simulink model "SixDOF_Equationgs_of_Motion"  (R2018a)
settings: Solver=VariableStepAuto  StartTime=0.0  StopTime=10  RelTol=1e-3
values from neighbouring files (symbols this model uses):
  CD0 = yD(find(~x))    [AOA_CL_CD_Cm.m]    (also in Linear_Coefficients.m = 0.051832)
  CDalpha = mean(diff(yD_linear)/d)    [AOA_CL_CD_Cm.m]    (also in Linear_Coefficients.m = 0.006587)
  CDdelta_e = 0.00036    [AOA_CL_CD_Cm.m]
  CL0 = yL(find(~x))    [AOA_CL_CD_Cm.m]    (also in Linear_Coefficients.m = 0.64791)
  CLalpha = mean(diff(yL_linear)/d)    [AOA_CL_CD_Cm.m]    (also in Linear_Coefficients.m = 0.088485)
  Clbeta = -0.00072    [AOA_CL_CD_Cm.m]    (also in Linear_Coefficients.m)
  Cldelta_a = -0.00393    [AOA_CL_CD_Cm.m]
  CLdelta_e = 0.00656    [AOA_CL_CD_Cm.m]    (also in Linear_Coefficients.m = 0.00328)
  Cldelta_r = -0.00008    (= -8e-05)    [AOA_CL_CD_Cm.m]
  Clp = -0.62    [AOA_CL_CD_Cm.m]    (also in Linear_Coefficients.m)
  Clr = -0.01    [AOA_CL_CD_Cm.m]    (also in Linear_Coefficients.m)
  Cm0 = ym(ZLI)    [AOA_CL_CD_Cm.m]    (also in Linear_Coefficients.m = -0.036061)
  Cmalpha = mean(diff(ym_linear)/d)    [AOA_CL_CD_Cm.m]    (also in Linear_Coefficients.m = -0.008902)
  Cmdelta_e = -0.01684    [AOA_CL_CD_Cm.m]    (also in Linear_Coefficients.m = -0.00842)
  Cnbeta = 0.00104    [AOA_CL_CD_Cm.m]    (also in Linear_Coefficients.m)
  Cndelta_a = 0.00034    [AOA_CL_CD_Cm.m]    (also in Linear_Coefficients.m)
  Cndelta_r = -0.00122    [AOA_CL_CD_Cm.m]    (also in Linear_Coefficients.m = -0.00061)
  Cnp = 0.004    [AOA_CL_CD_Cm.m]    (also in Linear_Coefficients.m)
  Cnr = -0.04    [AOA_CL_CD_Cm.m]    (also in Linear_Coefficients.m)
  CYbeta = -0.00668    [AOA_CL_CD_Cm.m]    (also in Linear_Coefficients.m)
  CYdelta_r = 0.00484    [AOA_CL_CD_Cm.m]    (also in Linear_Coefficients.m = 0.00242)
libraries: shared6dof x1, aerolibasang x1, aerolibatmos2 x1
settings Model: Creator=McQueen_Zero  LastModifiedBy=McQueen_Zero
settings DataIOCC: ExternalInput=[t, Alpha, delta_e, T, h, V, Beta, delta_r, delta_r]  LoadExternalInput=on

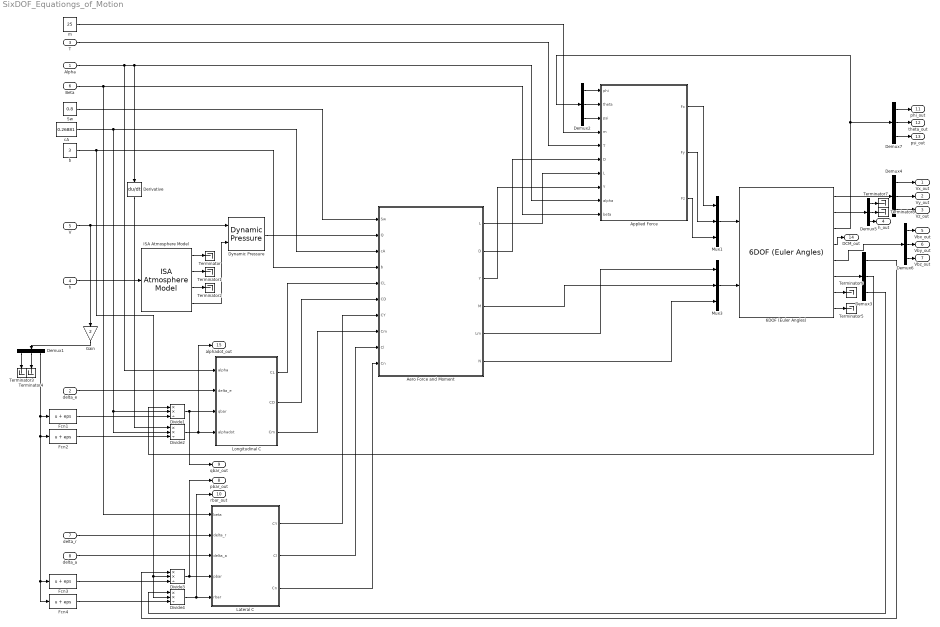
== system SixDOF_Equationgs_of_Motion ==
  Alpha : Inport
  delta_e : Inport  Port=2
  T : Inport  Port=3
  h : Inport  Port=4
  V : Inport  Port=5  PortDimensions=3
  Beta : Inport  Port=6
  delta_r : Inport  Port=7
  delta_a : Inport  Port=8
  6DOF (Euler Angles) : shared6dof/6DOF (Euler Angles)  units=Metric (MKS)  mtype=Fixed  rep=Euler Angles  xme_0=[0 0 0]  Vm_0=[25 0 0]  eul_0=[0 0 0]  pm_0=[0 0 0]  mass_0=25  mass_e=0.5  mass_f=2.0  inertia=eye(3)  inertia_e=eye(3)  inertia_f=2*eye(3)  k_quat=1.0  vre_flag=on  abi_flag=off  aMode=0
      settings: SourceProductBaseCode=AE
  Aero Force and Moment : Subsystem
  Applied Force : Subsystem
  Demux{1..7} (7 alike) : Demux  Outputs=3
  Derivative : Derivative
  Divide{1..4} (4 alike) : Product  Inputs=**/
  Dynamic Pressure : aerolibasang/Dynamic Pressure
  Fcn{1..4} (4 alike) : Fcn  Expr=u + eps
  Gain : Gain  Gain=2
  ISA Atmosphere Model : aerolibatmos2/ISA Atmosphere Model  custom=off  g=9.80665  gamma=1.4  R=287.0531  L=0.0065  h_trop=11000  h_strat=20000  rho0=1.225  P0=101325  T0=288.15  h0=0
      settings: SourceProductName=Aerospace Blockset
  Lateral C : Subsystem
  Longitudinal C : Subsystem
  Mux1 : Mux  Inputs=3
  Mux3 : Mux  Inputs=3
  Sw : Constant  Value=0.8
  Terminator{,1..5,7..9} (9 alike) : Terminator
  b : Constant  Value=3
  cA : Constant  Value=0.26881
  m : Constant  Value=25
  Vx_out : Outport
  Vy_out : Outport  Port=2
  Vz_out : Outport  Port=3
  h_out : Outport  Port=4
  Vbx_out : Outport  Port=5
  Vby_out : Outport  Port=6
  Vbz_out : Outport  Port=7
  pbar_out : Outport  Port=8
  qbar_out : Outport  Port=9
  rbar_out : Outport  Port=10
  phi_out : Outport  Port=11
  theta_out : Outport  Port=12
  psi_out : Outport  Port=13
  DCM_out : Outport  Port=14
  alphadot_out : Outport  Port=15
  wires:
  b/1 -> Divide3/2, Divide4/2, Aero Force and Moment/4(b)
  Longitudinal C/3(Cm) -> Aero Force and Moment/8(Cm)
  Divide2/1 -> alphadot_out/1, Longitudinal C/4(alphadot)
  Aero Force and Moment/6(N) -> Mux3/3
  Divide3/1 -> pbar_out/1, Lateral C/4(pbar)
  Divide1/1 -> qbar_out/1, Longitudinal C/3(qbar)
  Divide4/1 -> rbar_out/1, Lateral C/5(rbar)
  Demux3/3 -> Divide4/1
  Mux3/1 -> 6DOF (Euler Angles)/2
  Demux3/2 -> Divide1/1
  V/1 -> Dynamic Pressure/1, Gain/1
  Longitudinal C/2(CD) -> Aero Force and Moment/6(CD)
  Derivative/1 -> Divide2/1
  ISA Atmosphere Model/2 -> Terminator1/1
  Applied Force/1(Fx) -> Mux1/1
  Lateral C/1(CY) -> Aero Force and Moment/7(CY)
  Lateral C/2(Cl) -> Aero Force and Moment/9(Cl)
  delta_e/1 -> Longitudinal C/2(delta_e)
  delta_r/1 -> Lateral C/2(delta_r)
  Aero Force and Moment/2(D) -> Applied Force/6(D)
  h/1 -> ISA Atmosphere Model/1
  cA/1 -> Divide1/2, Divide2/2, Aero Force and Moment/3(cA)
  Lateral C/3(Cn) -> Aero Force and Moment/10(Cn)
  Longitudinal C/1(CL) -> Aero Force and Moment/5(CL)
  Aero Force and Moment/4(M) -> Mux3/2
  Demux3/1 -> Divide3/1
  ISA Atmosphere Model/4 -> Dynamic Pressure/2
  ISA Atmosphere Model/1 -> Terminator/1
  Dynamic Pressure/1 -> Aero Force and Moment/2(Q)
  ISA Atmosphere Model/3 -> Terminator2/1
  delta_a/1 -> Lateral C/3(delta_a)
  Applied Force/3(Fz) -> Mux1/3
  T/1 -> Applied Force/5(T)
  Aero Force and Moment/1(L) -> Applied Force/7(L)
  Aero Force and Moment/3(Y) -> Applied Force/8(Y)
  Sw/1 -> Aero Force and Moment/1(Sw)
  Beta/1 -> Lateral C/1(beta), Applied Force/10(beta)
  Alpha/1 -> Longitudinal C/1(alpha), Derivative/1, Applied Force/9(alpha)
  Applied Force/2(Fy) -> Mux1/2
  Mux1/1 -> 6DOF (Euler Angles)/1
  Aero Force and Moment/5(Lm) -> Mux3/1
  m/1 -> Applied Force/4(m)
  Demux2/1 -> Applied Force/1(phi)
  Demux2/2 -> Applied Force/2(theta)
  Demux2/3 -> Applied Force/3(psi)
  6DOF (Euler Angles)/6 -> Demux3/1
  Gain/1 -> Demux1/1
  Demux1/1 -> Terminator3/1
  Demux1/2 -> Terminator4/1
  6DOF (Euler Angles)/1 -> Demux4/1
  6DOF (Euler Angles)/2 -> Demux5/1
  6DOF (Euler Angles)/5 -> Demux6/1
  6DOF (Euler Angles)/7 -> Terminator9/1
  6DOF (Euler Angles)/8 -> Terminator5/1
  6DOF (Euler Angles)/4 -> DCM_out/1
  Demux4/1 -> Vx_out/1
  Demux4/2 -> Vy_out/1
  Demux4/3 -> Vz_out/1
  Demux5/1 -> Terminator7/1
  Demux5/2 -> Terminator8/1
  Demux5/3 -> h_out/1
  Demux6/1 -> Vbx_out/1
  Demux6/2 -> Vby_out/1
  Demux6/3 -> Vbz_out/1
  6DOF (Euler Angles)/3 -> Demux7/1, Demux2/1
  Demux7/1 -> phi_out/1
  Demux7/2 -> theta_out/1
  Demux7/3 -> psi_out/1
  Fcn3/1 -> Divide3/3
  Fcn4/1 -> Divide4/3
  Fcn2/1 -> Divide2/3
  Fcn1/1 -> Divide1/3
  Demux1/3 -> Fcn1/1, Fcn2/1, Fcn3/1, Fcn4/1

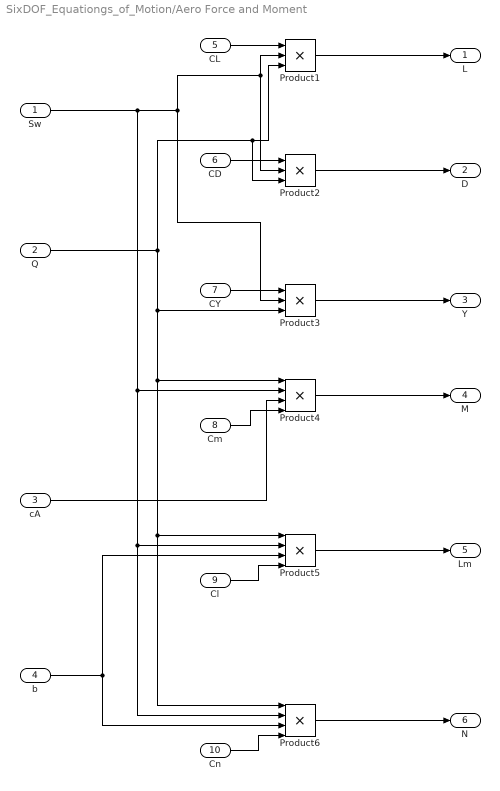
== system SixDOF_Equationgs_of_Motion/Aero Force and Moment ==
  Sw : Inport
  Q : Inport  Port=2
  cA : Inport  Port=3
  b : Inport  Port=4
  CL : Inport  Port=5
  CD : Inport  Port=6
  CY : Inport  Port=7
  Cm : Inport  Port=8
  Cl : Inport  Port=9
  Cn : Inport  Port=10
  Product1 : Product  Inputs=3
  Product2 : Product  Inputs=3
  Product3 : Product  Inputs=3
  Product4 : Product  Inputs=4
  Product5 : Product  Inputs=4
  Product6 : Product  Inputs=4
  L : Outport
  D : Outport  Port=2
  Y : Outport  Port=3
  M : Outport  Port=4
  Lm : Outport  Port=5
  N : Outport  Port=6
  wires:
  Sw/1 -> Product4/2, Product5/2, Product6/2, Product3/2, Product1/2, Product2/2
  Q/1 -> Product2/3, Product1/3, Product6/1, Product5/1, Product4/1, Product3/3
  b/1 -> Product6/3, Product5/3
  Cn/1 -> Product6/4
  cA/1 -> Product4/3
  CL/1 -> Product1/1
  Cm/1 -> Product4/4
  Product4/1 -> M/1
  Product2/1 -> D/1
  CD/1 -> Product2/1
  Cl/1 -> Product5/4
  Product3/1 -> Y/1
  Product6/1 -> N/1
  Product5/1 -> Lm/1
  CY/1 -> Product3/1
  Product1/1 -> L/1

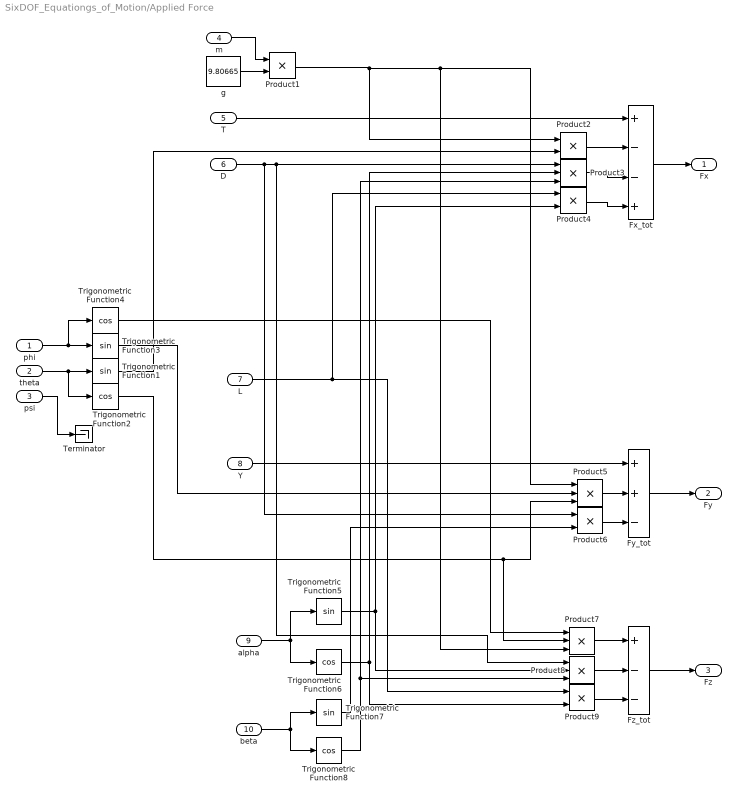
== system SixDOF_Equationgs_of_Motion/Applied Force ==
  phi : Inport
  theta : Inport  Port=2
  psi : Inport  Port=3
  m : Inport  Port=4
  T : Inport  Port=5
  D : Inport  Port=6
  L : Inport  Port=7
  Y : Inport  Port=8
  alpha : Inport  Port=9
  beta : Inport  Port=10
  Fx_tot : Sum  Inputs=+--+
  Fy_tot : Sum  Inputs=++-
  Fz_tot : Sum  Inputs=+--
  Product{1..2,4,6,9} (5 alike) : Product
  Product{3,5,7..8} (4 alike) : Product  Inputs=3
  Terminator : Terminator
  Trigonometric Function{1,3,5,7} (4 alike) : Trigonometry
  Trigonometric Function{2,4,6,8} (4 alike) : Trigonometry  Operator=cos
  g : Constant  Value=9.80665
  Fx : Outport
  Fy : Outport  Port=2
  Fz : Outport  Port=3
  wires:
  Trigonometric Function8/1 -> Product8/3, Product3/3
  L/1 -> Product9/1, Product4/1
  Trigonometric Function6/1 -> Product9/2, Product3/2
  Trigonometric Function5/1 -> Product8/2, Product4/2
  D/1 -> Product6/1, Product8/1, Product3/1
  Product1/1 -> Product7/3, Product5/1, Product2/1
  Product4/1 -> Fx_tot/4
  Trigonometric Function1/1 -> Product2/2
  alpha/1 -> Trigonometric Function6/1, Trigonometric Function5/1
  Trigonometric Function4/1 -> Product7/1
  Trigonometric Function2/1 -> Product5/3, Product7/2
  Product5/1 -> Fy_tot/2
  Trigonometric Function3/1 -> Product5/2
  T/1 -> Fx_tot/1
  phi/1 -> Trigonometric Function4/1, Trigonometric Function3/1
  theta/1 -> Trigonometric Function2/1, Trigonometric Function1/1
  g/1 -> Product1/2
  Product6/1 -> Fy_tot/3
  m/1 -> Product1/1
  Product9/1 -> Fz_tot/3
  beta/1 -> Trigonometric Function8/1, Trigonometric Function7/1
  Product8/1 -> Fz_tot/2
  Trigonometric Function7/1 -> Product6/2
  Product2/1 -> Fx_tot/2
  Product7/1 -> Fz_tot/1
  Product3/1 -> Fx_tot/3
  Y/1 -> Fy_tot/1
  psi/1 -> Terminator/1
  Fx_tot/1 -> Fx/1
  Fy_tot/1 -> Fy/1
  Fz_tot/1 -> Fz/1

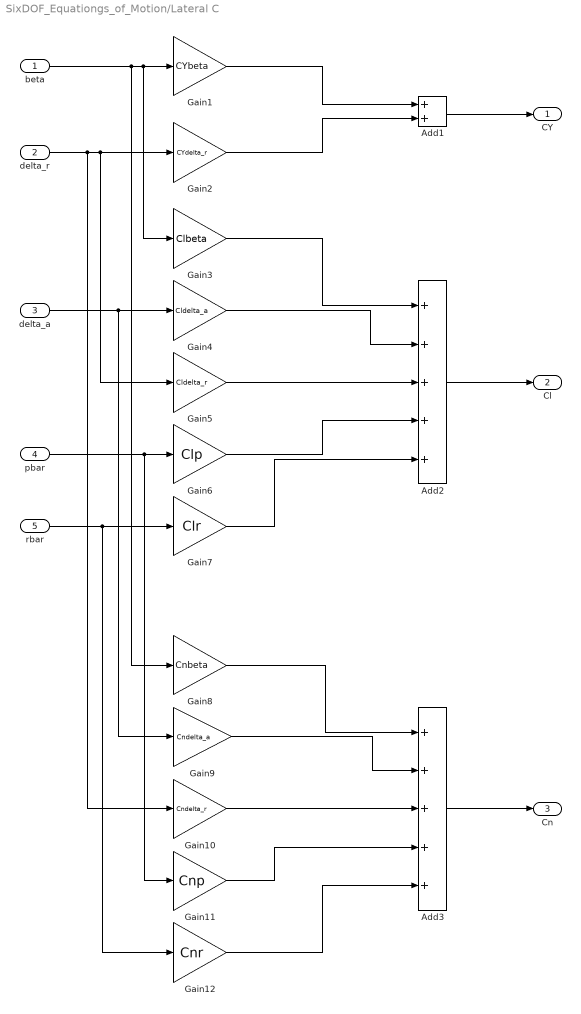
== system SixDOF_Equationgs_of_Motion/Lateral C ==
  beta : Inport
  delta_r : Inport  Port=2
  delta_a : Inport  Port=3
  pbar : Inport  Port=4
  rbar : Inport  Port=5
  Add1 : Sum
  Add2 : Sum  Inputs=+++++
  Add3 : Sum  Inputs=+++++
  Gain1 : Gain  Gain=CYbeta
  Gain10 : Gain  Gain=Cndelta_r
  Gain11 : Gain  Gain=Cnp
  Gain12 : Gain  Gain=Cnr
  Gain2 : Gain  Gain=CYdelta_r
  Gain3 : Gain  Gain=Clbeta
  Gain4 : Gain  Gain=Cldelta_a
  Gain5 : Gain  Gain=Cldelta_r
  Gain6 : Gain  Gain=Clp
  Gain7 : Gain  Gain=Clr
  Gain8 : Gain  Gain=Cnbeta
  Gain9 : Gain  Gain=Cndelta_a
  CY : Outport
  Cl : Outport  Port=2
  Cn : Outport  Port=3
  wires:
  delta_r/1 -> Gain10/1, Gain5/1, Gain2/1
  beta/1 -> Gain8/1, Gain3/1, Gain1/1
  Gain12/1 -> Add3/5
  Add3/1 -> Cn/1
  pbar/1 -> Gain11/1, Gain6/1
  Gain1/1 -> Add1/1
  delta_a/1 -> Gain9/1, Gain4/1
  Gain2/1 -> Add1/2
  Gain5/1 -> Add2/3
  Gain11/1 -> Add3/4
  rbar/1 -> Gain12/1, Gain7/1
  Add2/1 -> Cl/1
  Gain9/1 -> Add3/2
  Gain4/1 -> Add2/2
  Gain3/1 -> Add2/1
  Add1/1 -> CY/1
  Gain8/1 -> Add3/1
  Gain6/1 -> Add2/4
  Gain10/1 -> Add3/3
  Gain7/1 -> Add2/5

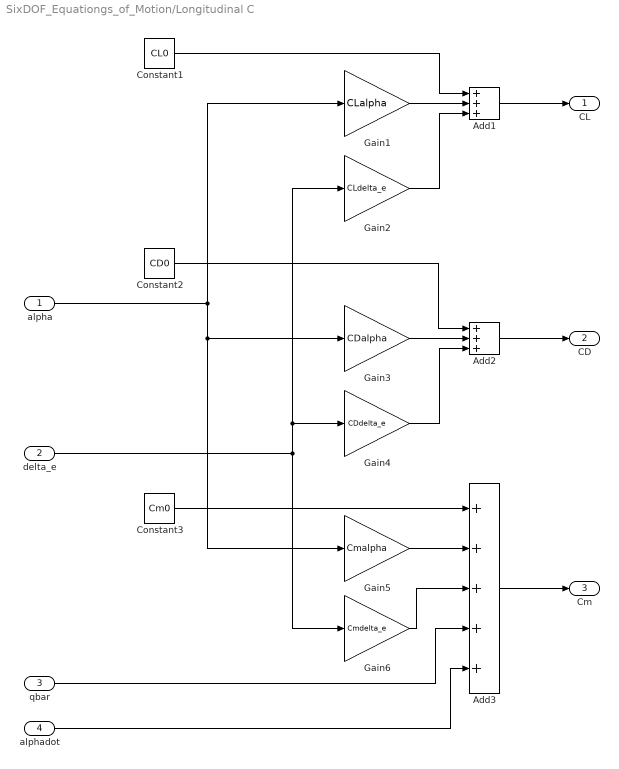
== system SixDOF_Equationgs_of_Motion/Longitudinal C ==
  alpha : Inport
  delta_e : Inport  Port=2
  qbar : Inport  Port=3
  alphadot : Inport  Port=4
  Add1 : Sum  Inputs=+++
  Add2 : Sum  Inputs=+++
  Add3 : Sum  Inputs=+++++
  Constant1 : Constant  Value=CL0
  Constant2 : Constant  Value=CD0
  Constant3 : Constant  Value=Cm0
  Gain1 : Gain  Gain=CLalpha
  Gain2 : Gain  Gain=CLdelta_e
  Gain3 : Gain  Gain=CDalpha
  Gain4 : Gain  Gain=CDdelta_e
  Gain5 : Gain  Gain=Cmalpha
  Gain6 : Gain  Gain=Cmdelta_e
  CL : Outport
  CD : Outport  Port=2
  Cm : Outport  Port=3
  wires:
  Add1/1 -> CL/1
  Constant1/1 -> Add1/1
  Constant2/1 -> Add2/1
  Gain3/1 -> Add2/2
  Add2/1 -> CD/1
  Constant3/1 -> Add3/1
  Gain4/1 -> Add2/3
  alphadot/1 -> Add3/5
  Gain1/1 -> Add1/2
  Add3/1 -> Cm/1
  alpha/1 -> Gain3/1, Gain5/1, Gain1/1
  delta_e/1 -> Gain6/1, Gain4/1, Gain2/1
  Gain2/1 -> Add1/3
  Gain5/1 -> Add3/2
  Gain6/1 -> Add3/3
  qbar/1 -> Add3/4
